simulink model "panda"  (R2022b)
settings: Solver=VariableStepAuto  StartTime=0.0  StopTime=10  EnableMultiTasking=on
values from neighbouring files (symbols this model uses):
  en = 1    [main_manipulator.m]
  q0 = [-pi/4 -3*pi/4]    [main_manipulator.m]
  q2 = [-0.785398163397 -0.78574787628 -0.786097014423 -0.786445577071 -0.786793563474 -0.787140972883 -0.787487804552 -0.787834057739 -0.788179731704 -0.788524825712 -0.78886933903 -0.789213270926 ... (6284 elements, 1x6284)]    [q2.mat]
  sr = 0.01    [main_manipulator.m]
  T = 1    [main_manipulator.m]
  w0 = 0.*[(q2(2)-q2(1))/(T/length(q2)) (q4(2)-q4(1))/(T/length(q4))]    [main_manipulator.m]
undefined symbols (not defined in the file or in its folder): Acceleration_1, Acceleration_2, Center_1, Center_2, magnitude, Pitch_1, Pitch_2, q4, Radius_1, Radius_2, Transformation_1, Transformation_2, tt, X, x_ee, Y, y_ee, Z
libraries: nesl_utility x15, sm_lib x14, simulink x14, slpidlib x4, franka_simulink_library x2, rllib x1
(part 2 of 2)

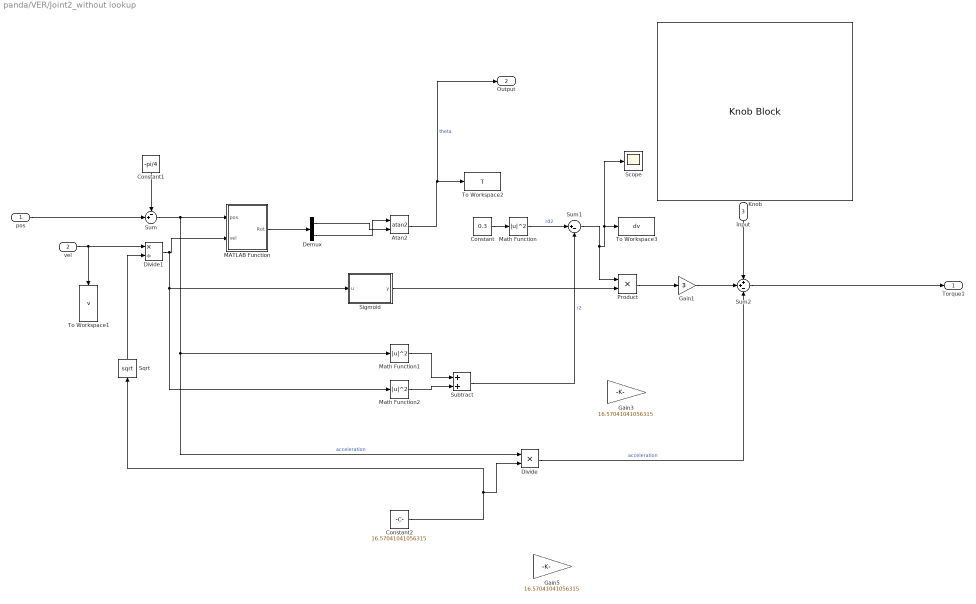
== system panda/VER/Joint2_without lookup ==
  pos : Inport
  vel : Inport  Port=2
  Input : Inport  Port=3
  Atan2 : Trigonometry  Operator=atan2
  Constant : Constant  Value=0.3
  Constant1 : Constant  Value=-pi/4
  Constant2 : Constant  Value=16.57041041056315
  Demux : Demux  Outputs=2
  Divide : Product  Inputs=**
  Divide1 : Product  Inputs=*/
  Gain1 : Gain  Gain=3
  Gain3 : Gain  Gain=16.57041041056315
  Gain5 : Gain  Gain=16.57041041056315
  Knob : KnobBlock  ScaleMax=3  TickInterval=0.10000000000000001
  MATLAB Function : MATLAB Function  TreatAsAtomicUnit=on
  Math Function : Math  Operator=magnitude^2  SignedPower=on
  Math Function1 : Math  Operator=magnitude^2  SignedPower=on
  Math Function2 : Math  Operator=magnitude^2  SignedPower=on
  Product : Product
  Scope : Scope
  Sigmoid : MATLAB Function  TreatAsAtomicUnit=on
  Sqrt : Sqrt
  Subtract : Sum
  Sum : Sum  Inputs=-+|
  Sum1 : Sum  Inputs=|+-
  Sum2 : Sum  Inputs=++-
  To Workspace1 : ToWorkspace  VariableName=v  SampleTime=-1
  To Workspace2 : ToWorkspace  VariableName=T  SampleTime=-1
  To Workspace3 : ToWorkspace  VariableName=dv  SampleTime=-1
  Torque1 : Outport  VectorParamsAs1DForOutWhenUnconnected=off
  Output : Outport  Port=2  VectorParamsAs1DForOutWhenUnconnected=off
  wires:
  Sqrt/1 -> Divide1/2
  Divide1/1 -> MATLAB Function/2(vel), Sigmoid/1(u), Math Function2/1
  vel/1 -> Divide1/1, To Workspace1/1
  Constant2/1 -> Divide/2, Sqrt/1
  Divide/1 -> Sum2/3  "acceleration"
  Demux/1 -> Atan2/2
  Sum/1 -> Math Function1/1, Divide/1, MATLAB Function/1(pos)  "acceleration"
  Subtract/1 -> Sum1/2  "r2"
  Demux/2 -> Atan2/1
  Atan2/1 -> To Workspace2/1, Output/1  "theta"
  Sum2/1 -> Torque1/1
  Math Function1/1 -> Subtract/1
  Math Function/1 -> Sum1/1  "rd2"
  Input/1 -> Sum2/1
  Gain1/1 -> Sum2/2
  Sum1/1 -> Scope/1, To Workspace3/1, Product/1
  Product/1 -> Gain1/1
  Constant1/1 -> Sum/1
  MATLAB Function/1(Rot) -> Demux/1
  Math Function2/1 -> Subtract/2
  Constant/1 -> Math Function/1
  pos/1 -> Sum/2
  Sigmoid/1(y) -> Product/2

== matlab function panda/C(q,dq)/MATLAB Function1 ==
  data: u input; y output
function y = fcn(u)

% l1 = 0.316;
% l2 = 0.2906;
l1 = 1;
l2 = 1;
m1 = 1;
m2 = 1;
g  = 0;

q1  = u(1);
dq1 = u(2);
q2  = u(4);
dq2 = u(5);
dx  = 0;
dy  = 0;
cg=[(m2*((dq1*l1*cos(q1) + (l2*cos(q1 + q2)*(dq1 + dq2))/2)*(2*dq1*l1*sin(q1) - 2*dx + l2*sin(q1 + q2)*(dq1 + dq2)) - (dq1*l1*sin(q1) + (l2*sin(q1 + q2)*(dq1 + dq2))/2)*(2*dy + 2*dq1*l1*cos(q1) + l2*cos(q1 + q2)*(dq1 + dq2)) - ((l2*cos(q1 + q2))/2 + l1*cos(q1))*(l2*sin(q1 + q2)*(dq1 + dq2)^2 + 2*dq1^2*l1*sin(q1)) + ((l2*sin(q1 + q2))/2 + l1*sin(q1))*(2*dq1^2*l1*cos(q1) + l2*cos(q1 + q2)*(dq1 + dq2)^2)))/2 - (m2*((dq1*l1*cos(q1) + (l2*cos(q1 + q2)*(dq1 + dq2))/2)*(2*dq1*l1*sin(q1) - 2*dx + l2*sin(q1 + q2)*(dq1 + dq2)) - (dq1*l1*sin(q1) + (l2*sin(q1 + q2)*(dq1 + dq2))/2)*(2*dy + 2*dq1*l1*cos(q1) + l2*cos(q1 + q2)*(dq1 + dq2))))/2 + g*m2*((l2*cos(q1 + q2))/2 + l1*cos(q1)) + (g*l1*m1*cos(q1))/2 ...
   ;                                                                                                                                                                   (m2*(l2*sin(q1 + q2)*(dq1^2*l1*cos(q1) + (l2*cos(q1 + q2)*(dq1 + dq2)^2)/2) - l2*cos(q1 + q2)*((l2*sin(q1 + q2)*(dq1 + dq2)^2)/2 + dq1^2*l1*sin(q1)) - l2*sin(q1 + q2)*(dq1 + dq2)*(dy + dq1*l1*cos(q1) + (l2*cos(q1 + q2)*(dq1 + dq2))/2) + l2*cos(q1 + q2)*(dq1 + dq2)*(dq1*l1*sin(q1) - dx + (l2*sin(q1 + q2)*(dq1 + dq2))/2)))/2 + (m2*(l2*sin(q1 + q2)*(dq1 + dq2)*(dy + dq1*l1*cos(q1) + (l2*cos(q1 + q2)*(dq1 + dq2))/2) - l2*cos(q1 + q2)*(dq1 + dq2)*(dq1*l1*sin(q1) - dx + (l2*sin(q1 + q2)*(dq1 + dq2))/2)))/2 + (g*l2*m2*cos(q1 + q2))/2 ...
   ;                                                                                                                                                                                                                                                                                                                                                                                                                                                                                                                                                                                                                                - (m2*(2*dq1^2*l1*cos(q1) + l2*cos(q1 + q2)*(dq1 + dq2)^2))/2 - (dq1^2*l1*m1*cos(q1))/2 ...
   ;                                                                                                                                                                                                                                                                                                                                                                                                                                                                                                                                                                                                                    g*m1 + g*m2 - (m2*(l2*sin(q1 + q2)*(dq1 + dq2)^2 + 2*dq1^2*l1*sin(q1)))/2 - (dq1^2*l1*m1*sin(q1))/2];


y = cg(1:2);

== matlab function panda/ARM/G/MATLAB Function1 ==
  data: u input; y output; fs output; bs1 input; bs2 input
function [y,fs] = fcn(u, bs1, bs2)

% bs = [0.23;0.83];
bs = [bs1; bs2];

l1 = 1;
l2 = 1;
m1 = 1;
m2 = 1;
d  = 0.1; 
g  = 9.81;

q1  = u(1);
dq1 = u(2)*0;
q2  = u(4);
dq2 = u(5)*0;
dx  = 0;
dy  = 0;

cg=[(m2*((dq1*l1*cos(q1) + (l2*cos(q1 + q2)*(dq1 + dq2))/2)*(2*dq1*l1*sin(q1) - 2*dx + l2*sin(q1 + q2)*(dq1 + dq2)) - (dq1*l1*sin(q1) + (l2*sin(q1 + q2)*(dq1 + dq2))/2)*(2*dy + 2*dq1*l1*cos(q1) + l2*cos(q1 + q2)*(dq1 + dq2)) - ((l2*cos(q1 + q2))/2 + l1*cos(q1))*(l2*sin(q1 + q2)*(dq1 + dq2)^2 + 2*dq1^2*l1*sin(q1)) + ((l2*sin(q1 + q2))/2 + l1*sin(q1))*(2*dq1^2*l1*cos(q1) + l2*cos(q1 + q2)*(dq1 + dq2)^2)))/2 - (m2*((dq1*l1*cos(q1) + (l2*cos(q1 + q2)*(dq1 + dq2))/2)*(2*dq1*l1*sin(q1) - 2*dx + l2*sin(q1 + q2)*(dq1 + dq2)) - (dq1*l1*sin(q1) + (l2*sin(q1 + q2)*(dq1 + dq2))/2)*(2*dy + 2*dq1*l1*cos(q1) + l2*cos(q1 + q2)*(dq1 + dq2))))/2 + g*m2*((l2*cos(q1 + q2))/2 + l1*cos(q1)) + (g*l1*m1*cos(q1))/2 ...
   ;                                                                                                                                                                   (m2*(l2*sin(q1 + q2)*(dq1^2*l1*cos(q1) + (l2*cos(q1 + q2)*(dq1 + dq2)^2)/2) - l2*cos(q1 + q2)*((l2*sin(q1 + q2)*(dq1 + dq2)^2)/2 + dq1^2*l1*sin(q1)) - l2*sin(q1 + q2)*(dq1 + dq2)*(dy + dq1*l1*cos(q1) + (l2*cos(q1 + q2)*(dq1 + dq2))/2) + l2*cos(q1 + q2)*(dq1 + dq2)*(dq1*l1*sin(q1) - dx + (l2*sin(q1 + q2)*(dq1 + dq2))/2)))/2 + (m2*(l2*sin(q1 + q2)*(dq1 + dq2)*(dy + dq1*l1*cos(q1) + (l2*cos(q1 + q2)*(dq1 + dq2))/2) - l2*cos(q1 + q2)*(dq1 + dq2)*(dq1*l1*sin(q1) - dx + (l2*sin(q1 + q2)*(dq1 + dq2))/2)))/2 + (g*l2*m2*cos(q1 + q2))/2 ...
   ;                                                                                                                                                                                                                                                                                                                                                                                                                                                                                                                                                                                                                                - (m2*(2*dq1^2*l1*cos(q1) + l2*cos(q1 + q2)*(dq1 + dq2)^2))/2 - (dq1^2*l1*m1*cos(q1))/2 ...
   ;                                                                                                                                                                                                                                                                                                                                                                                                                                                                                                                                                                                                                    g*m1 + g*m2 - (m2*(l2*sin(q1 + q2)*(dq1 + dq2)^2 + 2*dq1^2*l1*sin(q1)))/2 - (dq1^2*l1*m1*sin(q1))/2];

fs = - bs.*atan([u(2);u(5)]*100)*2/pi;


y  = cg(1:2) + fs;

== matlab function panda/VER/Dumble LC2/MATLAB Function ==
  data: pos input; Rot output; vel input
function Rot = fcn(pos, vel)

t0 = atan2(vel, pos);
Rotz = rotz(rad2deg(t0)); 
Rot = Rotz(1:2, 1:2) * [pos; vel];

== matlab function panda/Mass Matrix/Multiplay_Mass ==
  data: u input; y output
function y = fcn(u)

% l1 = 0.316;
% l2 = 0.2906;
l1 = 1;
l2 = 1;
m1 = 1;
m2 = 1;
d  = 0.1;

I1 = m1 * (l1^2 + d^2) /12;
I2 = m2 * (l2^2 + d^2) /12;

q1 = u(1);
q2 = u(4);

D=[I1 + I2 + (m2*((l2*cos(q1 + q2) + 2*l1*cos(q1))*((l2*cos(q1 + q2))/2 + l1*cos(q1)) + (l2*sin(q1 + q2) + 2*l1*sin(q1))*((l2*sin(q1 + q2))/2 + l1*sin(q1))))/2 + (m1*((l1^2*cos(q1)^2)/2 + (l1^2*sin(q1)^2)/2))/2, I2 + (m2*(l2*sin(q1 + q2)*((l2*sin(q1 + q2))/2 + l1*sin(q1)) + l2*cos(q1 + q2)*((l2*cos(q1 + q2))/2 + l1*cos(q1))))/2, - (m2*(l2*sin(q1 + q2) + 2*l1*sin(q1)))/2 - (l1*m1*sin(q1))/2, m2*((l2*cos(q1 + q2))/2 + l1*cos(q1)) + (l1*m1*cos(q1))/2 ...
  ;                                                                                           I2 + (m2*(l2*sin(q1 + q2)*((l2*sin(q1 + q2))/2 + l1*sin(q1)) + l2*cos(q1 + q2)*((l2*cos(q1 + q2))/2 + l1*cos(q1))))/2,                                                       I2 + (m2*((l2^2*cos(q1 + q2)^2)/2 + (l2^2*sin(q1 + q2)^2)/2))/2,                                       -(l2*m2*sin(q1 + q2))/2,                                    (l2*m2*cos(q1 + q2))/2 ...
  ;                                                                                                                                                   - (m2*(l2*sin(q1 + q2) + 2*l1*sin(q1)))/2 - (l1*m1*sin(q1))/2,                                                                                               -(l2*m2*sin(q1 + q2))/2,                                                       m1 + m2,                                                         0 ...
  ;                                                                                                                                                     (m2*(l2*cos(q1 + q2) + 2*l1*cos(q1)))/2 + (l1*m1*cos(q1))/2,                                                                                                (l2*m2*cos(q1 + q2))/2,                                                             0,                                                   m1 + m2];

y = D(1:2,1:2)*[u(7);u(8)];

== matlab function panda/VER/Dumble LC2/Sigmoid ==
  data: u input; y output
function y = fcn(u)

% y = 2 * (1./(1+exp(-u)) - 0.5);
y=sign(u);

end

== matlab function panda/PD/MATLAB Function ==
  data: X input; Q2 output; Y input; Q4 output
function [Q2, Q4]= InverseKinematics(X, Y)
%    l1 = sqrt(0.316^2+0.088^2);
%    l2 = sqrt(0.384^2+0.088^2);
    l1 = 1;
    l2 = 1;
    
    Q4 = -(pi-acos((-X.^2 - Y.^2 + l1.^2 + l2.^2)./(2.*l1.*l2)));
    Q2 =  atan2((l2.*sin(Q4)), (l2.*cos(Q4)+l1)) - atan2(X, Y);
end

== matlab function panda/VER/Joint2_without lookup/MATLAB Function ==
  data: pos input; Rot output; vel input
function Rot = fcn(pos, vel)

t0 = atan2(vel, pos);
Rotz = rotz(rad2deg(t0)); 
Rot = Rotz(1:2, 1:2) * [pos; vel];

== matlab function panda/VER/Joint2_without lookup/Sigmoid ==
  data: u input; y output
function y = fcn(u)

% y = 2 * (1./(1+exp(-u)) - 0.5);
y=u;

end

== matlab function panda/VER/Joint2 with lookup1/MATLAB Function ==
  data: pos input; Rot output; vel input
function Rot = fcn(pos, vel)

t0 = atan2(vel, pos);
Rotz = rotz(rad2deg(t0)); 
Rot = Rotz(1:2, 1:2) * [pos; vel];

== matlab function panda/VER/Joint2 with lookup1/Sigmoid ==
  data: u input; y output
function y = fcn(u)

% y = 2 * (1./(1+exp(-u)) - 0.5);
y=u;

end
